simulink model "take_off_flag"  (R2018a)
settings: Solver=ode1  StartTime=0.0  StopTime=10.0  FixedStep=T  RelTol=1e-3  EnableMultiTasking=on
undefined symbols (not defined in the file): X0
settings Model: Creator=ahmad  LastModifiedBy=ahmad
settings OptimizationCC: LifeSpan=inf
settings DebuggingCC: SFUnexpectedBacktrackingDiag=warning  SFNoUnconditionalDefaultTransitionDiag=warning  SFExecutionAtInitializationDiag=none
settings CodeAppCC: StateflowObjectComments=on
settings GRTTargetCC: TargetLangStandard=C89/C90 (ANSI)  GeneratePreprocessorConditionals=Disable all
settings ConfigComp: CovMetricSettings=dw  CovHtmlReporting=on  CovSaveCumulativeToWorkspaceVar=on  CovSaveSingleToWorkspaceVar=on  CovExternalEMLEnable=off

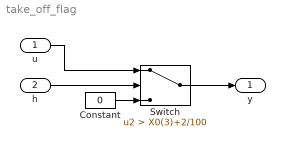
== system take_off_flag ==
  u : Inport
  h : Inport  Port=2
  Constant : Constant  Value=0
  Switch : Switch  Criteria=u2 > Threshold  Threshold=X0(3)+2/100
  y : Outport
  wires:
  u/1 -> Switch/1
  h/1 -> Switch/2
  Constant/1 -> Switch/3
  Switch/1 -> y/1
